simulink model "untitled"  (R2015b)
settings: Solver=VariableStepAuto  StartTime=0.0  StopTime=inf  RelTol=1e-3
libraries: arduino_io_lib x3
settings Model: Creator=Xavier  LastModifiedBy=Xavier

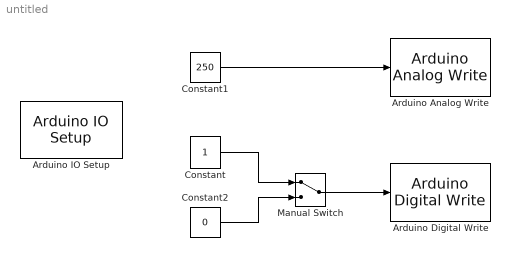
== system untitled ==
  Arduino Analog Write : arduino_io_lib/Arduino Analog Write  arduinoVar=Arduino1  arduinoPin=9  T=0.2
  Arduino Digital Write : arduino_io_lib/Arduino Digital Write  arduinoVar=Arduino1  arduinoPin=8  T=0.2
  Arduino IO Setup : arduino_io_lib/Arduino IO Setup  Priority=3  arduinoVar=Arduino1  comPort=COM3
  Constant : Constant
  Constant1 : Constant  Value=250
  Constant2 : Constant  Value=0
  Manual Switch : ManualSwitch
  wires:
  Constant1/1 -> Arduino Analog Write/1
  Manual Switch/1 -> Arduino Digital Write/1
  Constant/1 -> Manual Switch/1
  Constant2/1 -> Manual Switch/2
